simulink model "AUAV_V3_TestSensors"  (R2015a)
settings: Solver=FixedStepDiscrete  StartTime=0.0  StopTime=10.0  FixedStep=T  RelTol=1e-3
PreLoadFcn:
  | %T = 0.0025;
  | MavlinkBus;
  | mcuInit;
  | % Baro Altitude Computation
  | % =========================
  | basePressure = 98192.64;
  | baseTemp = 288.215;
  | lapseRate = -0.00198122;
  | baseHeight = 0;
values from neighbouring files (symbols this model uses):
  apSampleTime = 0.01    [mcuInit.m]
  latlong_WP = 1    [mcuInit.m]
  mavlink_attitude_t = Simulink.Bus    [MavlinkBusMarcello.m]
  mavlink_gps_raw_int_t = Simulink.Bus    [MavlinkBus.m]    (also in MavlinkBusMarcello.m)
  mavlink_raw_imu_t = Simulink.Bus    [MavlinkBus.m]    (also in MavlinkBusMarcello.m)
  mavlink_scaled_pressure_t = Simulink.Bus    [MavlinkBus.m]    (also in MavlinkBusMarcello.m)
  mavlink_servo_output_raw_t = Simulink.Bus    [MavlinkBusMarcello.m]
  mavlink_slugs_navigation_t = Simulink.Bus    [MavlinkBusMarcello.m]
  mavlink_sys_status_t = Simulink.Bus    [MavlinkBus.m]    (also in MavlinkBusMarcello.m)
  T = 0.01    [mcuInit.m]
  Xpoints = [0 0]    [mcuInit.m]
  Ypoints = [0 0]    [mcuInit.m]
  Zpoints = [0 0]    [mcuInit.m]
undefined symbols (not defined in the file or in its folder): A0, A14, A15, A2, A3, A4, A5, A6, accBiasRateLimit, B0, bankCommandLimit, barAdjust, baroCutoff, baroCutTemp, cubeAccelGain16405, cubeGyroGain16405, cubeMagGain16405, D0, D11, D7, D8, daLimit, data, daTrimMax, daTrimMin, deLimit, deTrimMax, deTrimMin, drLimit, drTrimMax, drTrimMin, dtLimit, dtTrimMax, dtTrimMin, F2, F3, G0, G13, G15, gaind, GS_location, gyroBiasRateLimit, IC1max, IPStar, ISA_g, Max, maxAcc, MaxDwnPthStar, maxDynPressure, maxEta, mlParamInterface, ms, OC1max, P112, P125, P127, P16, P20, P21, P30 ... (+26)
undefined symbols (not defined in the file): baroOffset, baroScale, barTGain1, barTGain2, barTMean1, barTMean2, bda, bde, bdr, bdt, bICda, bICde, bICdr, bICdt, derivativesConstant, lowRateSensorCutoff, mainSensorCutoff, mda, mde, mdr, mdt, mICda, mICde, mICdr, mICdt, pitotOffset, pitotScale, pitTGain1, pitTGain2, pitTMean1, pitTMean2, powerOffset, powerScale, pressureSensorCutoff, tempOffset, tempScale, vzCutoff, xCutoff, yCutoff
libraries: MCHP_Blockset x158, simulink x84, SLUGS_Library x31, aerolibconvert2 x6, aerolibutil x4, aerolibtransform2 x3, dspmtrx3 x2, aerolibobsolete x2
(part 24 of 24)

== matlab function AUAV_V3_TestSensors/Sensor_Data_Adapter/Sensor Suite/Low Pass Filtering,Temperature Compensation and Calibration/Tustin Lowpass, Auto Initial Condition2/Embedded MATLAB Function ==
  data: u input; y output; T input; f input
function y = fcn(u,T,f)
% This block supports an embeddable subset of the MATLAB language.
% See the help menu for details. 

persistent a
persistent b
persistent y_km1
persistent u_km1
if isempty(a)
    %tf = [T*omega/(2+T*omega) T*omega/(2+T*omega)],[1 (T*omega-2)/(T*omega+2)]
    %tf = [a a],[1 -b]
    omega = 2*pi*f;
    a=T*omega/(2+T*omega);
    b=-(T*omega-2)/(T*omega+2);
    y_km1=u;
    u_km1=u;
end

y = a*(u+u_km1)+b*y_km1;
y_km1=y;
u_km1=u;

== matlab function AUAV_V3_TestSensors/Sensor_Data_Adapter/Sensor Suite/Low Pass Filtering,Temperature Compensation and Calibration/Tustin Lowpass, Auto Initial Condition3/Embedded MATLAB Function ==
  data: u input; y output; T input; f input
function y = fcn(u,T,f)
% This block supports an embeddable subset of the MATLAB language.
% See the help menu for details. 

persistent a
persistent b
persistent y_km1
persistent u_km1
if isempty(a)
    %tf = [T*omega/(2+T*omega) T*omega/(2+T*omega)],[1 (T*omega-2)/(T*omega+2)]
    %tf = [a a],[1 -b]
    omega = 2*pi*f;
    a=T*omega/(2+T*omega);
    b=-(T*omega-2)/(T*omega+2);
    y_km1=u;
    u_km1=u;
end

y = a*(u+u_km1)+b*y_km1;
y_km1=y;
u_km1=u;

== matlab function AUAV_V3_TestSensors/Sensor_Data_Adapter/Sensor Suite/Low Pass Filtering,Temperature Compensation and Calibration/Tustin Lowpass, Auto Initial Condition4/Embedded MATLAB Function ==
  data: u input; y output; T input; f input
function y = fcn(u,T,f)
% This block supports an embeddable subset of the MATLAB language.
% See the help menu for details. 

persistent a
persistent b
persistent y_km1
persistent u_km1
if isempty(a)
    %tf = [T*omega/(2+T*omega) T*omega/(2+T*omega)],[1 (T*omega-2)/(T*omega+2)]
    %tf = [a a],[1 -b]
    omega = 2*pi*f;
    a=T*omega/(2+T*omega);
    b=-(T*omega-2)/(T*omega+2);
    y_km1=u;
    u_km1=u;
end

y = a*(u+u_km1)+b*y_km1;
y_km1=y;
u_km1=u;

== matlab function AUAV_V3_TestSensors/Inner Loop// Navigation/Navigation Encaps [updated 4.28.16]/Navigation/Circle Navigation/Intersection. Circular Navigation/Compute Angle Between Vectors2/negprotect3 ==
  data: val input; zpVal output
function zpVal = negProt(val)
% This block supports an embeddable subset of the MATLAB language.
% See the help menu for details. 

if val >= single(0.0001)
    zpVal = val;
else
    zpVal = single(0.0001);
end

== matlab function AUAV_V3_TestSensors/Inner Loop// Navigation/Navigation Encaps [updated 4.28.16]/Navigation/Circle Navigation/Intersection. Circular Navigation/Embedded MATLAB Function ==
  data: hFact input; P31 output; P2 input; P32 output
function [P31,P32] = getP3s(hFact, P2)
% This block supports an embeddable subset of the MATLAB language.
% See the help menu for details. 

P31 = single([0 0 0]');
P32 = single([0 0 0]');

P31(1) = P2(1) + hFact(2);
P32(1) = P2(1) - hFact(2);

P31(2) = P2(2) - hFact(1);
P32(2) = P2(2) + hFact(1);

== matlab function AUAV_V3_TestSensors/Inner Loop// Navigation/Navigation Encaps [updated 4.28.16]/Navigation/Circle Navigation/Intersection. Circular Navigation/dsPIC_SQRT/negprotect ==
  data: val input; zpVal output
function zpVal = negProt(val)
% This block supports an embeddable subset of the MATLAB language.
% See the help menu for details. 

if val >= single(0.001)
    zpVal = val;
else
    zpVal = single(0.001);
end

== matlab function AUAV_V3_TestSensors/Inner Loop// Navigation/Navigation Encaps [updated 4.28.16]/Navigation/Circle Navigation/Intersection. Circular Navigation/negprotect1 ==
  data: val input; zpVal output
function zpVal = negProt(val)
% This block supports an embeddable subset of the MATLAB language.
% See the help menu for details. 

if val >= single(0.0001)
    zpVal = val;
else
    zpVal = single(0.0001);
end

== matlab function AUAV_V3_TestSensors/Inner Loop// Navigation/Navigation Encaps [updated 4.28.16]/Navigation/Circle Navigation/Intersection. Circular Navigation/negprotect2 ==
  data: val input; zpVal output
function zpVal = negProt(val)
% This block supports an embeddable subset of the MATLAB language.
% See the help menu for details. 

if val >= single(0.0001)
    zpVal = val;
else
    zpVal = single(0.0001);
end

== matlab function AUAV_V3_TestSensors/Inner Loop// Navigation/Navigation Encaps [updated 4.28.16]/Navigation/Circle Navigation/Vector Norm/dsPIC_SQRT/negprotect ==
  data: val input; zpVal output
function zpVal = negProt(val)
% This block supports an embeddable subset of the MATLAB language.
% See the help menu for details. 

if val >= single(0.001)
    zpVal = val;
else
    zpVal = single(0.001);
end

== matlab function AUAV_V3_TestSensors/Inner Loop// Navigation/Navigation Encaps [updated 4.28.16]/Navigation/Get 2D Groundspeed/Vector Norm/dsPIC_SQRT/negprotect ==
  data: val input; zpVal output
function zpVal = negProt(val)
% This block supports an embeddable subset of the MATLAB language.
% See the help menu for details. 

if val >= single(0.001)
    zpVal = val;
else
    zpVal = single(0.001);
end

== matlab function AUAV_V3_TestSensors/Inner Loop// Navigation/Navigation Encaps [updated 4.28.16]/Navigation/L2+/Get Sin, Cos eta/Get Groundspeed/Vector Norm/dsPIC_SQRT/negprotect ==
  data: val input; zpVal output
function zpVal = negProt(val)
% This block supports an embeddable subset of the MATLAB language.
% See the help menu for details. 

if val >= single(0.001)
    zpVal = val;
else
    zpVal = single(0.001);
end

== matlab function AUAV_V3_TestSensors/Inner Loop// Navigation/Navigation Encaps [updated 4.28.16]/Navigation/L2+/Get Sin, Cos eta/Get Groundspeed/Zero out Z1 ==
  data: P output; Pin input
function P = P2D(Pin)
% This block supports an embeddable subset of the MATLAB language.
% See the help menu for details. 

P = [Pin(1); Pin(2); 0];

== matlab function AUAV_V3_TestSensors/Inner Loop// Navigation/Navigation Encaps [updated 4.28.16]/Navigation/L2+/Get Sin, Cos eta/negprotect ==
  data: val input; zpVal output
function zpVal = negProt(val)
% This block supports an embeddable subset of the MATLAB language.
% See the help menu for details. 

if val >= single(0.0001)
    zpVal = val;
else
    zpVal = single(0.0001);
end

== matlab function AUAV_V3_TestSensors/Inner Loop// Navigation/Navigation Encaps [updated 4.28.16]/Navigation/L2+/L2+/negprotect ==
  data: val input; zpVal output
function zpVal = negProt(val)
% This block supports an embeddable subset of the MATLAB language.
% See the help menu for details. 

if val >= single(0.0001)
    zpVal = val;
else
    zpVal = single(0.0001);
end

== matlab function AUAV_V3_TestSensors/Inner Loop// Navigation/Navigation Encaps [updated 4.28.16]/Navigation/Line Segment/Vector Norm/dsPIC_SQRT/negprotect ==
  data: val input; zpVal output
function zpVal = negProt(val)
% This block supports an embeddable subset of the MATLAB language.
% See the help menu for details. 

if val >= single(0.001)
    zpVal = val;
else
    zpVal = single(0.001);
end

== matlab function AUAV_V3_TestSensors/Inner Loop// Navigation/Navigation Encaps [updated 4.28.16]/Navigation/Normal WP Navigation/Compute WP Switching Trigger/dsPIC_SQRT/negprotect ==
  data: val input; zpVal output
function zpVal = negProt(val)
% This block supports an embeddable subset of the MATLAB language.
% See the help menu for details. 

if val >= single(0.001)
    zpVal = val;
else
    zpVal = single(0.001);
end

== matlab function AUAV_V3_TestSensors/Inner Loop// Navigation/Navigation Encaps [updated 4.28.16]/Navigation/Normal WP Navigation/Embedded MATLAB Function ==
  data: wpEnable input; reached output; didReachIP input
function reached = didUAVReachIp(wpEnable, didReachIP)
% This functions keeps track if the IP has been reached and if so
% it disables homing of IP until WP is reset

persistent persistentDidReachIP;


% initialize the persistent and the return value to 1
% so WP, and not homing, is active by default
if isempty(persistentDidReachIP)
    persistentDidReachIP =  uint8(0);
end


% this is just turned on for one sample 
% inmediatley upon enabling the navigation.
% Reset the flag the the IP was reached
if wpEnable
    persistentDidReachIP = uint8(0);
end

% Once the IP is reached the the persistent variable
% preserves the values until reset
if didReachIP
    persistentDidReachIP = uint8(1);
end;

reached = persistentDidReachIP;

== matlab function AUAV_V3_TestSensors/Inner Loop// Navigation/Navigation Encaps [updated 4.28.16]/Navigation/Normal WP Navigation/Get Frenet/Compute Frenet/Normalize Vector/Vector Norm/dsPIC_SQRT/negprotect ==
  data: val input; zpVal output
function zpVal = negProt(val)
% This block supports an embeddable subset of the MATLAB language.
% See the help menu for details. 

if val >= single(0.001)
    zpVal = val;
else
    zpVal = single(0.001);
end

== matlab function AUAV_V3_TestSensors/Inner Loop// Navigation/Navigation Encaps [updated 4.28.16]/Navigation/Normal WP Navigation/Get Frenet/Zero out Z1 ==
  data: P output; Pin input
function P = P2D(Pin)
% This block supports an embeddable subset of the MATLAB language.
% See the help menu for details. 

P = [Pin(1); Pin(2); 0];

== matlab function AUAV_V3_TestSensors/Inner Loop// Navigation/Navigation Encaps [updated 4.28.16]/Navigation/Normal WP Navigation/Get Frenet/Zero out Z2 ==
  data: P output; Pin input
function P = P2D(Pin)
% This block supports an embeddable subset of the MATLAB language.
% See the help menu for details. 

P = [Pin(1); Pin(2); 0];

== matlab function AUAV_V3_TestSensors/Inner Loop// Navigation/Navigation Encaps [updated 4.28.16]/Navigation/Normal WP Navigation/Get Frenet/Zero out Z3 ==
  data: P output; Pin input
function P = P2D(Pin)
% This block supports an embeddable subset of the MATLAB language.
% See the help menu for details. 

P = [Pin(1); Pin(2); 0];

== matlab function AUAV_V3_TestSensors/Inner Loop// Navigation/Navigation Encaps [updated 4.28.16]/Navigation/Normal WP Navigation/Zero out Z2 ==
  data: P output; Pin input
function P = P2D(Pin)
% This block supports an embeddable subset of the MATLAB language.
% See the help menu for details. 

P = [Pin(1); Pin(2); 0];

== matlab function AUAV_V3_TestSensors/Inner Loop// Navigation/Navigation Encaps [updated 4.28.16]/Navigation/Normal WP Navigation/computeCurrentWP ==
  data: WPSwitch input; maxWp input; IPReached input; WP0 output; WP1 output
function [WP0,WP1] = computeCurrentWP(WPSwitch, maxWp, IPReached)
% This functions keeps track if the IP has been reached and if so
% it disables homing of IP until WP is reset

persistent fromWp;
persistent toWp;

% initialize the persistent and the return value to 1
% so WP, and not homing, is active by default
if isempty(fromWp)
    fromWp =  uint8(1);
    toWp = uint8(2);
end

if WPSwitch
    fromWp = toWp;
    toWp = toWp +1;
    if (toWp > maxWp)
        toWp = uint8(1);
    end
end


% this is jturned on long as we have not reached IP 
if ~IPReached
    fromWp = uint8(1);
    toWp = uint8(2);
end



WP0 = fromWp;
WP1 = toWp;

== matlab function AUAV_V3_TestSensors/Inner Loop// Navigation/Navigation Encaps [updated 4.28.16]/Navigation/RTB//Follow Mobile Navigation/Zero out Z1 ==
  data: P output; Pin input
function P = P2D(Pin)
% This block supports an embeddable subset of the MATLAB language.
% See the help menu for details. 

P = [Pin(1); Pin(2); 0];

== matlab function AUAV_V3_TestSensors/Inner Loop// Navigation/Navigation Encaps [updated 4.28.16]/Navigation/Zero out Z1 ==
  data: P output; Pin input
function P = P2D(Pin)
% This block supports an embeddable subset of the MATLAB language.
% See the help menu for details. 

P = [Pin(1); Pin(2); 0];

== matlab function AUAV_V3_TestSensors/Inner Loop// Navigation/Navigation Encaps [updated 4.28.16]/Navigation/Zero out Z2 ==
  data: P output; Pin input
function P = P2D(Pin)
% This block supports an embeddable subset of the MATLAB language.
% See the help menu for details. 

P = [Pin(1); Pin(2); 0];

== matlab function AUAV_V3_TestSensors/Inner Loop// Navigation/Navigation Encaps [updated 4.28.16]/Navigation/myMux Fun1 ==
  data: u1 input; y output; u2 input; u3 input; u4 input
function y = FeedNavNavAcordingToMode(u1, u2, u3, u4)
% This block supports an embeddable subset of the MATLAB language.
% See the help menu for details. 
y = [u1(1); u2(1); u3(1); u4(1)];

== matlab function AUAV_V3_TestSensors/Inner Loop// Navigation/Navigation Encaps [updated 4.28.16]/Navigation/myMux Fun2 ==
  data: u1 input; y output; u2 input; u3 input
function y = myMux(u1, u2, u3)
% This block supports an embeddable subset of the MATLAB language.
% See the help menu for details. 

y = [u1(1); u2(1); u3(1)];

== matlab function AUAV_V3_TestSensors/Inner Loop// Navigation/Navigation Encaps [updated 4.28.16]/Navigation/myMux Fun3 ==
  data: u1 input; y output; u2 input
function y = myMux(u1, u2)
% This block supports an embeddable subset of the MATLAB language.
% See the help menu for details. 

y = [u1(1); u1(2); u2(1)];

== matlab function AUAV_V3_TestSensors/Inner Loop// Navigation/Navigation Encaps [updated 4.28.16]/Navigation/myMux Fun4 ==
  data: u1 input; y output; u2 input; u3 input
function y = myMux(u1, u2, u3)
% This block supports an embeddable subset of the MATLAB language.
% See the help menu for details. 

y = [u1(1); u2(1); u3(1)];

== matlab function AUAV_V3_TestSensors/Inner Loop// Navigation/Navigation Encaps [updated 4.28.16]/Navigation/myMux Fun5 ==
  data: u1 input; y output; u2 input; u3 input
function y = myMux(u1, u2, u3)
% This block supports an embeddable subset of the MATLAB language.
% See the help menu for details. 

y = [u1(1); u2(1); u3(1)];

== matlab function AUAV_V3_TestSensors/Inner Loop// Navigation/Navigation Encaps [updated 4.28.16]/Navigation/myMux Fun6 ==
  data: u1 input; y output; u2 input; u3 input
function y = myMux(u1, u2, u3)
% This block supports an embeddable subset of the MATLAB language.
% See the help menu for details. 

y = [u1(1); u2(1); u3(1)];

== matlab function AUAV_V3_TestSensors/Trim Vals [updated 4.28.16]/Bufffer IC/Buffer IC Channel ==
  data: latest input; history output
function history = bufferICValues(latest)
% This block supports an embeddable subset of the MATLAB language.
% See the help menu for details. 

persistent oldValues;

if isempty(oldValues)
    oldValues = uint16([0 0 0 0 0 0 0]);
end

history = uint16([0 0 0 0 0 0 0]);

for i=7:-1:2
    oldValues(i) = oldValues(i-1);
	history(i) = oldValues(i-1);
end
	
oldValues(1) = latest;
history(1) = latest;

== matlab function AUAV_V3_TestSensors/Trim Vals [updated 4.28.16]/Bufffer IC/Buffer IC Channel1 ==
  data: latest input; history output
function history = bufferICValues(latest)
% This block supports an embeddable subset of the MATLAB language.
% See the help menu for details. 

persistent oldValues;

if isempty(oldValues)
    oldValues = uint16([0 0 0 0 0 0 0]);
end

history = uint16([0 0 0 0 0 0 0]);

for i=7:-1:2
    oldValues(i) = oldValues(i-1);
	history(i) = oldValues(i-1);
end
	
oldValues(1) = latest;
history(1) = latest;

== matlab function AUAV_V3_TestSensors/Trim Vals [updated 4.28.16]/Bufffer IC/Buffer IC Channel2 ==
  data: latest input; history output
function history = bufferICValues(latest)
% This block supports an embeddable subset of the MATLAB language.
% See the help menu for details. 

persistent oldValues;

if isempty(oldValues)
    oldValues = uint16([0 0 0 0 0 0 0]);
end

history = uint16([0 0 0 0 0 0 0]);

for i=7:-1:2
    oldValues(i) = oldValues(i-1);
	history(i) = oldValues(i-1);
end
	
oldValues(1) = latest;
history(1) = latest;

== matlab function AUAV_V3_TestSensors/Trim Vals [updated 4.28.16]/Bufffer IC/Buffer IC Channel3 ==
  data: latest input; history output
function history = bufferICValues(latest)
% This block supports an embeddable subset of the MATLAB language.
% See the help menu for details. 

persistent oldValues;

if isempty(oldValues)
    oldValues = uint16([0 0 0 0 0 0 0]);
end

history = uint16([0 0 0 0 0 0 0]);

for i=7:-1:2
    oldValues(i) = oldValues(i-1);
	history(i) = oldValues(i-1);
end
	
oldValues(1) = latest;
history(1) = latest;

== matlab function AUAV_V3_TestSensors/Trim Vals [updated 4.28.16]/Control Surface Input/2 sec  tau/Embedded MATLAB Function ==
  data: u input; y output; T input; f input
function y = fcn(u,T,f)
% This block supports an embeddable subset of the MATLAB language.
% See the help menu for details. 

persistent a
persistent b
persistent y_km1
persistent u_km1
if isempty(a)
    %tf = [T*omega/(2+T*omega) T*omega/(2+T*omega)],[1 (T*omega-2)/(T*omega+2)]
    %tf = [a a],[1 -b]
    omega = 2*pi*f;
    a=T*omega/(2+T*omega);
    b=-(T*omega-2)/(T*omega+2);
    y_km1=u;
    u_km1=u;
end

y = a*(u+u_km1)+b*y_km1;
y_km1=y;
u_km1=u;

== matlab function AUAV_V3_TestSensors/Trim Vals [updated 4.28.16]/Control Surface Input/2 sec  tau1/Embedded MATLAB Function ==
  data: u input; y output; T input; f input
function y = fcn(u,T,f)
% This block supports an embeddable subset of the MATLAB language.
% See the help menu for details. 

persistent a
persistent b
persistent y_km1
persistent u_km1
if isempty(a)
    %tf = [T*omega/(2+T*omega) T*omega/(2+T*omega)],[1 (T*omega-2)/(T*omega+2)]
    %tf = [a a],[1 -b]
    omega = 2*pi*f;
    a=T*omega/(2+T*omega);
    b=-(T*omega-2)/(T*omega+2);
    y_km1=u;
    u_km1=u;
end

y = a*(u+u_km1)+b*y_km1;
y_km1=y;
u_km1=u;

== matlab function AUAV_V3_TestSensors/Trim Vals [updated 4.28.16]/Control Surface Input/myMux Fun1 ==
  data: u1 input; y output; u2 input
function y = myMux(u1, u2)
% This block supports an embeddable subset of the MATLAB language.
% See the help menu for details. 

y = [u1(1); u2(1)];

== matlab function AUAV_V3_TestSensors/Trim Vals [updated 4.28.16]/Control Surface Input/myMux Fun5 ==
  data: u1 input; y output; u2 input; u3 input; u4 input; u5 input
function y = myMux(u1, u2, u3, u4, u5)
% This block supports an embeddable subset of the MATLAB language.
% See the help menu for details. 

y = [u1(1); u2(1); u3(1); u4(1); u5(1)];

== matlab function AUAV_V3_TestSensors/Trim Vals [updated 4.28.16]/Mean Filter the Transition/Buffer Failsafe Channel ==
  data: latest input; history output
function history = bufferICValues(latest)
% This block supports an embeddable subset of the MATLAB language.
% See the help menu for details. 

persistent oldValues;

if isempty(oldValues)
    oldValues = uint16([0 0 0 0 0 0 0]);
end

history = uint16([0 0 0 0 0 0 0]);

for i=7:-1:2
    oldValues(i) = oldValues(i-1);
	history(i) = oldValues(i-1);
end
	
oldValues(1) = latest;
history(1) = latest;

== matlab function AUAV_V3_TestSensors/Update PWM Commands and Send Telemetry [updated 4.27.16]/Generate PWM Signals Based on the Control Type/If  Control Type Is Selective Passthrough/myMux Fun1 ==
  data: u1 input; y output; u2 input; u3 input; u4 input
function y = myMux(u1, u2, u3, u4 )
% This block supports an embeddable subset of the MATLAB language.
% See the help menu for details. 

y = [u1(1); u2(1); u3(1); u4(1)];

== matlab function AUAV_V3_TestSensors/Update PWM Commands and Send Telemetry [updated 4.27.16]/Generate PWM Signals Based on the Control Type/If  Control Type Is Wp, ISR, LP or  Mid Lvl Cmds/myMux Fun1 ==
  data: u1 input; y output; u2 input; u3 input; u4 input
function y = myMux(u1, u2, u3, u4 )
% This block supports an embeddable subset of the MATLAB language.
% See the help menu for details. 

y = [u1(1); u2(1); u3(1); u4(1)];

== matlab function AUAV_V3_TestSensors/get Nav Vars [updated 4.28.16]/Embedded MATLAB Function1 ==
  data: u input; y output
function y = TwoPi(u)
% This block supports an embeddable subset of the MATLAB language.
% See the help menu for details. 

if ( u < 0 )
    y = u + 2*pi;
else
    y = u;
end

== matlab function AUAV_V3_TestSensors/get Nav Vars [updated 4.28.16]/myMux Fun1 ==
  data: u1 input; y output; u2 input; u3 input
function y = myMux3(u1, u2, u3)
% This block supports an embeddable subset of the MATLAB language.
% See the help menu for details. 

y = [u1(1); u2(1); u3(1)];

== matlab function AUAV_V3_TestSensors/Inner Loop// Navigation/Navigation Encaps [updated 4.28.16]/Navigation/Normal WP Navigation/Get Frenet/Compute Frenet/Select N Terms ==
  data: T input; N output
function N = getN(T)
% This block supports an embeddable subset of the MATLAB language.
% See the help menu for details. 

N = [-T(2); T(1); 0];

== matlab function AUAV_V3_TestSensors/Inner Loop// Navigation/Navigation Encaps [updated 4.28.16]/Navigation/Normal WP Navigation/Get Frenet/Compute Frenet/Normalize Vector /Vector Norm/dsPIC_SQRT/negprotect ==
  data: val input; zpVal output
function zpVal = negProt(val)
% This block supports an embeddable subset of the MATLAB language.
% See the help menu for details. 

if val >= single(0.001)
    zpVal = val;
else
    zpVal = single(0.001);
end

== matlab function AUAV_V3_TestSensors/Inner Loop// Navigation/Navigation Encaps [updated 4.28.16]/Navigation/Normal WP Navigation/Get Frenet/get WP Coord from Index1/Get WP from idx SIM/Zero out Z1 ==
  data: y output; idx input; vect input
function y = GetVectorElement(idx , vect)
% This block supports an embeddable subset of the MATLAB language.
% See the help menu for details. 

y = vect(idx);

== matlab function AUAV_V3_TestSensors/Inner Loop// Navigation/Navigation Encaps [updated 4.28.16]/Navigation/Normal WP Navigation/Get Frenet/get WP Coord from Index1/Get WP from idx SIM/Zero out Z2 ==
  data: y output; idx input; vect input
function y = GetVectorElement(idx , vect)
% This block supports an embeddable subset of the MATLAB language.
% See the help menu for details. 

y = vect(idx);

== matlab function AUAV_V3_TestSensors/Inner Loop// Navigation/Navigation Encaps [updated 4.28.16]/Navigation/Normal WP Navigation/Get Frenet/get WP Coord from Index1/Get WP from idx SIM/Zero out Z3 ==
  data: y output; idx input; vect input
function y = GetVectorElement(idx , vect)
% This block supports an embeddable subset of the MATLAB language.
% See the help menu for details. 

y = vect(idx);

== matlab function AUAV_V3_TestSensors/Inner Loop// Navigation/Navigation Encaps [updated 4.28.16]/Navigation/Normal WP Navigation/Get Frenet/get WP Coord from Index2/Get WP from idx SIM/Zero out Z1 ==
  data: y output; idx input; vect input
function y = GetVectorElement(idx , vect)
% This block supports an embeddable subset of the MATLAB language.
% See the help menu for details. 

y = vect(idx);

== matlab function AUAV_V3_TestSensors/Inner Loop// Navigation/Navigation Encaps [updated 4.28.16]/Navigation/Normal WP Navigation/Get Frenet/get WP Coord from Index2/Get WP from idx SIM/Zero out Z2 ==
  data: y output; idx input; vect input
function y = GetVectorElement(idx , vect)
% This block supports an embeddable subset of the MATLAB language.
% See the help menu for details. 

y = vect(idx);

== matlab function AUAV_V3_TestSensors/Inner Loop// Navigation/Navigation Encaps [updated 4.28.16]/Navigation/Normal WP Navigation/Get Frenet/get WP Coord from Index2/Get WP from idx SIM/Zero out Z3 ==
  data: y output; idx input; vect input
function y = GetVectorElement(idx , vect)
% This block supports an embeddable subset of the MATLAB language.
% See the help menu for details. 

y = vect(idx);

== matlab function AUAV_V3_TestSensors/Inner Loop// Navigation/Navigation Encaps [updated 4.28.16]/Navigation/Normal WP Navigation/On WP Enable/Subsystem/Compute Frenet/Normalize Vector/Vector Norm/dsPIC_SQRT/negprotect ==
  data: val input; zpVal output
function zpVal = negProt(val)
% This block supports an embeddable subset of the MATLAB language.
% See the help menu for details. 

if val >= single(0.001)
    zpVal = val;
else
    zpVal = single(0.001);
end

== matlab function AUAV_V3_TestSensors/Inner Loop// Navigation/Navigation Encaps [updated 4.28.16]/Navigation/Normal WP Navigation/On WP Enable/Subsystem/Compute Frenet/Select N Terms ==
  data: T input; N output
function N = getN(T)
% This block supports an embeddable subset of the MATLAB language.
% See the help menu for details. 

N = [-T(2); T(1); 0];

== matlab function AUAV_V3_TestSensors/Inner Loop// Navigation/Navigation Encaps [updated 4.28.16]/Navigation/Normal WP Navigation/On WP Enable/Subsystem/Compute Frenet/Normalize Vector /Vector Norm/dsPIC_SQRT/negprotect ==
  data: val input; zpVal output
function zpVal = negProt(val)
% This block supports an embeddable subset of the MATLAB language.
% See the help menu for details. 

if val >= single(0.001)
    zpVal = val;
else
    zpVal = single(0.001);
end

== matlab function AUAV_V3_TestSensors/Inner Loop// Navigation/Navigation Encaps [updated 4.28.16]/Navigation/Normal WP Navigation/On WP Enable/Subsystem/get WP Coord from Index/Get WP from idx SIM/Zero out Z1 ==
  data: y output; idx input; vect input
function y = GetVectorElement(idx , vect)
% This block supports an embeddable subset of the MATLAB language.
% See the help menu for details. 

y = vect(idx);

== matlab function AUAV_V3_TestSensors/Inner Loop// Navigation/Navigation Encaps [updated 4.28.16]/Navigation/Normal WP Navigation/On WP Enable/Subsystem/get WP Coord from Index/Get WP from idx SIM/Zero out Z2 ==
  data: y output; idx input; vect input
function y = GetVectorElement(idx , vect)
% This block supports an embeddable subset of the MATLAB language.
% See the help menu for details. 

y = vect(idx);

== matlab function AUAV_V3_TestSensors/Inner Loop// Navigation/Navigation Encaps [updated 4.28.16]/Navigation/Normal WP Navigation/On WP Enable/Subsystem/get WP Coord from Index/Get WP from idx SIM/Zero out Z3 ==
  data: y output; idx input; vect input
function y = GetVectorElement(idx , vect)
% This block supports an embeddable subset of the MATLAB language.
% See the help menu for details. 

y = vect(idx);

== matlab function AUAV_V3_TestSensors/Inner Loop// Navigation/Navigation Encaps [updated 4.28.16]/Navigation/Normal WP Navigation/On WP Enable/Subsystem/get WP Coord from Index1/Get WP from idx SIM/Zero out Z1 ==
  data: y output; idx input; vect input
function y = GetVectorElement(idx , vect)
% This block supports an embeddable subset of the MATLAB language.
% See the help menu for details. 

y = vect(idx);

== matlab function AUAV_V3_TestSensors/Inner Loop// Navigation/Navigation Encaps [updated 4.28.16]/Navigation/Normal WP Navigation/On WP Enable/Subsystem/get WP Coord from Index1/Get WP from idx SIM/Zero out Z2 ==
  data: y output; idx input; vect input
function y = GetVectorElement(idx , vect)
% This block supports an embeddable subset of the MATLAB language.
% See the help menu for details. 

y = vect(idx);

== matlab function AUAV_V3_TestSensors/Inner Loop// Navigation/Navigation Encaps [updated 4.28.16]/Navigation/Normal WP Navigation/On WP Enable/Subsystem/get WP Coord from Index1/Get WP from idx SIM/Zero out Z3 ==
  data: y output; idx input; vect input
function y = GetVectorElement(idx , vect)
% This block supports an embeddable subset of the MATLAB language.
% See the help menu for details. 

y = vect(idx);

== matlab function AUAV_V3_TestSensors/Inner Loop// Navigation/Navigation Encaps [updated 4.28.16]/Navigation/Normal WP Navigation/Vector Norm/dsPIC_SQRT/negprotect ==
  data: val input; zpVal output
function zpVal = negProt(val)
% This block supports an embeddable subset of the MATLAB language.
% See the help menu for details. 

if val >= single(0.001)
    zpVal = val;
else
    zpVal = single(0.001);
end

== matlab function AUAV_V3_TestSensors/Inner Loop// Navigation/Navigation Encaps [updated 4.28.16]/Navigation/RTB//Follow Mobile Navigation/Vector Norm/dsPIC_SQRT/negprotect ==
  data: val input; zpVal output
function zpVal = negProt(val)
% This block supports an embeddable subset of the MATLAB language.
% See the help menu for details. 

if val >= single(0.001)
    zpVal = val;
else
    zpVal = single(0.001);
end

== matlab function AUAV_V3_TestSensors/get Nav Vars [updated 4.28.16]/myMux Fun2 ==
  data: u1 input; y output; u2 input
function y = myMux3(u1, u2)
% This block supports an embeddable subset of the MATLAB language.
% See the help menu for details. 

y = [u1(1:3); u2(1:3)];

== matlab function AUAV_V3_TestSensors/myMux Fun1 ==
  data: u1 input; y output; u2 input; u3 input; u4 input
function y = myMux(u1, u2, u3, u4 )
% This block supports an embeddable subset of the MATLAB language.
% See the help menu for details. 

y = [u1(1); u2(1); u3(1); u4(1)];

== matlab function AUAV_V3_TestSensors/Sensor_Data_Adapter/Raw HIL Readings/Enabled Subsystem1/Embedded MATLAB Function1 ==
  data: u input; y output
function y = averageADC(u)
% This block supports an embeddable subset of the MATLAB language.
% See the help menu for details. 

y = (u(1)+ u(2) + u(3) + u(4) + u(5))*0.20;

== matlab function AUAV_V3_TestSensors/Sensor_Data_Adapter/Raw HIL Readings/Enabled Subsystem1/Embedded MATLAB Function2 ==
  data: u input; y output
function y = averageADC(u)
% This block supports an embeddable subset of the MATLAB language.
% See the help menu for details. 

y = (u(1)+ u(2) + u(3) + u(4) + u(5))*0.20;

== matlab function AUAV_V3_TestSensors/Sensor_Data_Adapter/Raw HIL Readings/Enabled Subsystem1/myMux Fun ==
  data: u1 input; y output; u2 input; u3 input; u4 input
function y = myMux(u1, u2, u3, u4)
% This block supports an embeddable subset of the MATLAB language.
% See the help menu for details. 

y = [u1(1); u2(1); u3(1); u4(1)];
